simulink model "AB_Final_of_MPC_Bandwidth_Result_UnbalancedNew"  (R2022b)
settings: Solver=FixedStepDiscrete  StartTime=0.0  StopTime=Inf  FixedStep=100e-6  RelTol=1e-3  EnableMultiTasking=on
undefined symbols (not defined in the file): C28x, CPU1, CPU2, CurrentBypassValue, DiscIntNeverNeededParam, Down, GPTRIP1SEL, TZ1, Up
libraries: c2802xlib x20, simulink x17, dspstat3 x13, eeGeneralControl x10, c2837xDlib x5, c280xlib x5, PID_Lib x4, c2000lib x1, spsAlphaBetaZerotoabcLib x1
(part 3 of 10)

== system AB_Final_of_MPC_Bandwidth_Result_UnbalancedNew/Subsystem3 ==
  MPCC_f32GridVoltageA2 : Inport
  MPCC_f32GridVoltageB1 : Inport  Port=2
  MPCC_f32GridVoltageC3 : Inport  Port=3
  function : TriggerPort  TriggerType=function-call  VariantControl=(inherit)
  Add5 : Sum  Inputs=+--
  Cast To Single{,1..4} (5 alike) : DataTypeConversion  OutDataTypeStr=single  SaturateOnIntegerOverflow=off  RndMeth=Floor
  Constant10 : Constant  Value=boolean(0)
  Constant11 : Constant  Value=single(56539)
  Constant12 : Constant  Value=single(100e-6)
  Constant13 : Constant  Value=boolean(0)
  Constant14 : Constant  Value=single(56539)
  Constant15 : Constant  Value=single(100e-6)
  Constant16 : Constant  Value=boolean(0)
  Constant3 : Constant  Value=single(56539)
  Constant4 : Constant  Value=single(100e-6)
  Constant5 : Constant  Value=single(0)
  Constant8 : Constant  Value=36000
  Gain{2,4,8,10} (4 alike) : Gain  Gain=-1
  Gain11 : Gain  Gain=single(1/0.85)
  Gain6 : Gain  Gain=single(1/0.9)
  Gain7 : Gain  Gain=single(1/0.9)
  LPF : Subsystem
  LPF1 : Subsystem
  LPF2 : Subsystem
  PLL_Loop2 : Subsystem
  Rate Limiter Dynamic : simulink/Discontinuities/Rate Limiter Dynamic
  RateLimiter : Subsystem
  RateLimiter1 : Subsystem
  RateLimiter2 : Subsystem
  MPCC_f32AngularFrequency : Outport
  MPCC_f32GridVoltageC : Outport  Port=2
  MPCC_f32ElectricalAngle : Outport  Port=3
  MPCC_f32GridVoltageA : Outport  Port=4
  MPCC_f32GridVoltageB : Outport  Port=5
  wires:
  Cast To Single1/1 -> Gain6/1
  Constant5/1 -> Add5/1
  Cast To Single2/1 -> Gain7/1
  LPF/1(y_k) -> Cast To Single1/1
  LPF2/1(y_k) -> Cast To Single2/1
  Gain7/1 -> Add5/3, PLL_Loop2/2(MPCC_f32GridVoltageB), MPCC_f32GridVoltageB/1
  MPCC_f32GridVoltageA2/1 -> RateLimiter/5(Xo), RateLimiter/4(U), Rate Limiter Dynamic/2
  Constant8/1 -> Gain8/1, Rate Limiter Dynamic/1
  Gain8/1 -> Rate Limiter Dynamic/3
  Constant3/1 -> Gain2/1, RateLimiter/1(Up)
  Gain2/1 -> RateLimiter/3(Lo)
  Constant4/1 -> RateLimiter/2(Ts)
  Constant10/1 -> RateLimiter/6(Rs)
  RateLimiter/1(Y) -> LPF/1(u_k)
  Constant11/1 -> Gain4/1, RateLimiter1/1(Up)
  Constant12/1 -> RateLimiter1/2(Ts)
  Gain4/1 -> RateLimiter1/3(Lo)
  MPCC_f32GridVoltageB1/1 -> RateLimiter1/5(Xo), RateLimiter1/4(U)
  Constant13/1 -> RateLimiter1/6(Rs)
  RateLimiter1/1(Y) -> LPF2/1(u_k)
  RateLimiter2/1(Y) -> LPF1/1(u_k)
  Constant16/1 -> RateLimiter2/6(Rs)
  Gain10/1 -> RateLimiter2/3(Lo)
  Constant15/1 -> RateLimiter2/2(Ts)
  Constant14/1 -> Gain10/1, RateLimiter2/1(Up)
  LPF1/1(y_k) -> Cast To Single4/1
  Cast To Single4/1 -> Gain11/1
  MPCC_f32GridVoltageC3/1 -> RateLimiter2/5(Xo), RateLimiter2/4(U)
  Gain11/1 -> PLL_Loop2/3(MPCC_f32GridVoltageC), MPCC_f32GridVoltageC/1
  PLL_Loop2/1(MPCC_f32AngularFrequency) -> Cast To Single/1
  Gain6/1 -> PLL_Loop2/1(MPCC_f32GridVoltageA), MPCC_f32GridVoltageA/1, Add5/2
  PLL_Loop2/2(MPCC_f32ElectricalAngle) -> Cast To Single3/1
  Cast To Single/1 -> MPCC_f32AngularFrequency/1
  Cast To Single3/1 -> MPCC_f32ElectricalAngle/1

== system AB_Final_of_MPC_Bandwidth_Result_UnbalancedNew/Subsystem4 ==
  function : TriggerPort  TriggerType=function-call  VariantControl=(inherit)
  Constant : Constant  Value=boolean(0)
  Digital Output : c2837xDlib/Digital Output  GPIO_Number=GPIO8~GPIO15  GPIO_Bit0=off  GPIO_BIT0_Toggle=off  GPIO_Bit1=off  GPIO_BIT1_Toggle=off  GPIO_Bit2=off  GPIO_BIT2_Toggle=off  GPIO_Bit3=off  GPIO_BIT3_Toggle=off  GPIO_Bit4=off  GPIO_BIT4_Toggle=off  GPIO_Bit5=off  GPIO_BIT5_Toggle=off  GPIO_Bit6=on  GPIO_BIT6_Toggle=off  GPIO_Bit7=off  GPIO_BIT7_Toggle=off
  wires:
  Constant/1 -> Digital Output/1

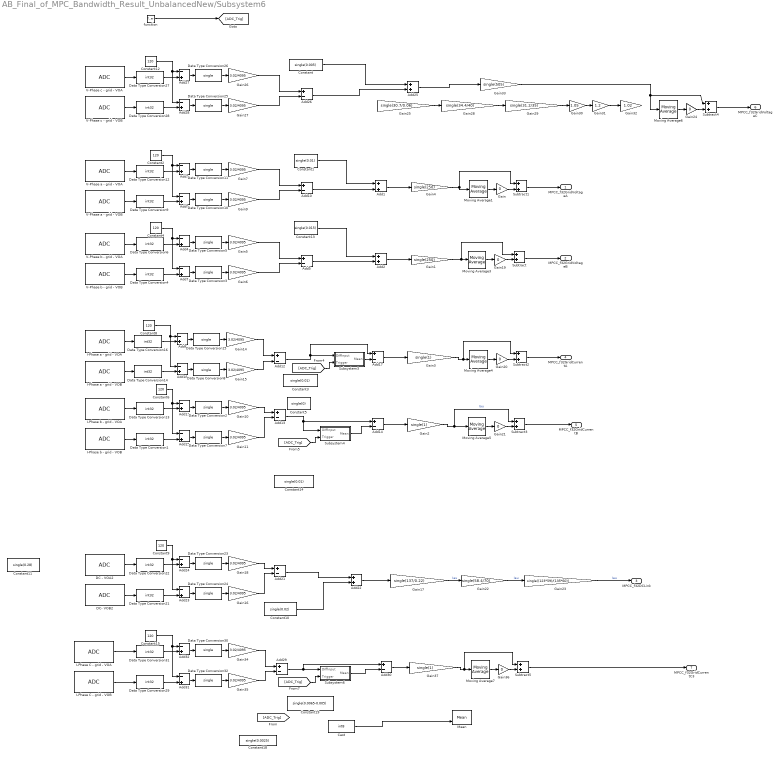
== system AB_Final_of_MPC_Bandwidth_Result_UnbalancedNew/Subsystem6 ==
  function : TriggerPort  TriggerType=function-call  VariantControl=(inherit)  ShowOutputPort=on  OutputDataType=int8
  Add{1..2,22,25} (4 alike) : Sum  AccumDataTypeStr=single  OutDataTypeStr=single
  Add{5,10,12..14,17,21,26,29..30} (10 alike) : Sum  Inputs=+-  AccumDataTypeStr=single  OutDataTypeStr=single
  Add{3..4,6..7,9,11,15,18,23..24,27..28,31..32} (14 alike) : Sum  Inputs=-+  AccumDataTypeStr=single  OutDataTypeStr=single
  Cast : DataTypeConversion  OutDataTypeStr=int8  SaturateOnIntegerOverflow=off  RndMeth=Floor
  Constant : Constant  Value=single(0.005)
  Constant1 : Constant  Value=single(0.01)
  Constant10 : Constant  Value=single(0.02)
  Constant11 : Constant  Value=single(0.28)
  Constant{2,4,6,8..9,12,15} (7 alike) : Constant  Value=120  OutDataTypeStr=single
  Constant13 : Constant  Value=single(0.015)
  Constant14 : Constant  Value=single(0.01)
  Constant18 : Constant  Value=single(0.0025)
  Constant19 : Constant  Value=single(0.0065-0.005)
  Constant3 : Constant  Value=single(0.01)
  Constant5 : Constant  Value=single(0)
  DC - VOA2 : c2802xlib/ADC  blkParamProc=C2000_Type4  ADCModule=C  samplingMode=Single sample mode  ADCResolution=12-bit (Single-ended input)  useSOC1=SOC0  useSOC2=SOC0_SOC1  SOCAcquisitionWindow=22  SOCTriggerSource=ePWM1_ADCSOCA  SOCInterruptTrigger=No ADCINT  Ts=-1  dType=uint16  postInterrupt=off  interruptSel=ADCINT1  ADCINTContinuous=on  endma=off  chdma=1  conv1=ADCINA0  conv2=ADCINA0 and ADCINB0  conv1_Type4=ADCIN5  conv2_Type4=ADCIN0 and ADCIN1
  DC- VOB2 : c2802xlib/ADC  blkParamProc=C2000_Type4  ADCModule=B  samplingMode=Single sample mode  ADCResolution=12-bit (Single-ended input)  useSOC1=SOC3  useSOC2=SOC0_SOC1  SOCAcquisitionWindow=22  SOCTriggerSource=ePWM1_ADCSOCA  SOCInterruptTrigger=No ADCINT  Ts=-1  dType=uint16  postInterrupt=off  interruptSel=ADCINT2  ADCINTContinuous=on  endma=off  chdma=1  conv1=ADCINA0  conv2=ADCINA0 and ADCINB0  conv1_Type4=ADCIN5  conv2_Type4=ADCIN2 and ADCIN3
  Data Type Conversion{1,4,6,9,12..14,16,21..22,27..29,31} (14 alike) : DataTypeConversion  OutDataTypeStr=int32  ConvertRealWorld=Stored Integer (SI)  SaturateOnIntegerOverflow=off  RndMeth=Floor
  Data Type Conversion{2..3,5,7..8,10..11,15,23..26,30,32} (14 alike) : DataTypeConversion  OutDataTypeStr=single  SaturateOnIntegerOverflow=off  RndMeth=Floor
  Gain{,19..21,24,36} (6 alike) : Gain  Gain=0
  Gain1 : Gain  Gain=single(250)
  Gain{5..7,9..11,14..16,18,26..27,34..35} (14 alike) : Gain  Gain=3.02/4095  ParamDataTypeStr=single  OutDataTypeStr=single
  Gain17 : Gain  Gain=single(137/0.22)
  Gain2 : Gain  Gain=single(1)
  Gain22 : Gain  Gain=single(58.4/70)
  Gain23 : Gain  Gain=single((123*59)/(135*60))
  Gain25 : Gain  Gain=single(30.7/0.06)
  Gain28 : Gain  Gain=single(34.4/40)
  Gain29 : Gain  Gain=single(31.2/35)
  Gain3 : Gain  Gain=single(1)
  Gain30 : Gain  Gain=1.05
  Gain31 : Gain  Gain=1.2
  Gain32 : Gain  Gain=1.02
  Gain33 : Gain  Gain=single(505)
  Gain37 : Gain  Gain=single(1)
  Gain4 : Gain  Gain=single(250)
  I-Phase C - grid - VOA : c2802xlib/ADC  blkParamProc=C2000_Type4  ADCModule=A  samplingMode=Single sample mode  ADCResolution=12-bit (Single-ended input)  useSOC1=SOC15  useSOC2=SOC0_SOC1  SOCAcquisitionWindow=22  SOCTriggerSource=ePWM1_ADCSOCA  SOCInterruptTrigger=No ADCINT  Ts=-1  dType=uint16  postInterrupt=off  interruptSel=ADCINT1  ADCINTContinuous=on  endma=off  chdma=1  conv1=ADCINA0  conv2=ADCINA0 and ADCINB0  conv1_Type4=ADCIN15  conv2_Type4=ADCIN0 and ADCIN1
  I-Phase C - grid - VOB : c2802xlib/ADC  blkParamProc=C2000_Type4  ADCModule=A  samplingMode=Single sample mode  ADCResolution=12-bit (Single-ended input)  useSOC1=SOC10  useSOC2=SOC0_SOC1  SOCAcquisitionWindow=22  SOCTriggerSource=ePWM1_ADCSOCA  SOCInterruptTrigger=No ADCINT  Ts=-1  dType=uint16  postInterrupt=off  interruptSel=ADCINT2  ADCINTContinuous=on  endma=off  chdma=1  conv1=ADCINA0  conv2=ADCINA0 and ADCINB0  conv1_Type4=ADCIN14  conv2_Type4=ADCIN2 and ADCIN3
  I-Phase a - grid - VOA : c2802xlib/ADC  blkParamProc=C2000_Type4  ADCModule=A  samplingMode=Single sample mode  ADCResolution=12-bit (Single-ended input)  useSOC1=SOC0  useSOC2=SOC0_SOC1  SOCAcquisitionWindow=22  SOCTriggerSource=ePWM1_ADCSOCA  SOCInterruptTrigger=No ADCINT  Ts=-1  dType=uint16  postInterrupt=on  interruptSel=ADCINT1  ADCINTContinuous=on  endma=off  chdma=1  conv1=ADCINA0  conv2=ADCINA0 and ADCINB0  conv1_Type4=ADCIN4  conv2_Type4=ADCIN0 and ADCIN1
  I-Phase a - grid - VOB : c2802xlib/ADC  blkParamProc=C2000_Type4  ADCModule=B  samplingMode=Single sample mode  ADCResolution=12-bit (Single-ended input)  useSOC1=SOC1  useSOC2=SOC0_SOC1  SOCAcquisitionWindow=22  SOCTriggerSource=ePWM1_ADCSOCA  SOCInterruptTrigger=No ADCINT  Ts=-1  dType=uint16  postInterrupt=off  interruptSel=ADCINT2  ADCINTContinuous=on  endma=off  chdma=1  conv1=ADCINA0  conv2=ADCINA0 and ADCINB0  conv1_Type4=ADCIN4  conv2_Type4=ADCIN2 and ADCIN3
  I-Phase b - grid - VOA : c2802xlib/ADC  blkParamProc=C2000_Type4  ADCModule=C  samplingMode=Single sample mode  ADCResolution=12-bit (Single-ended input)  useSOC1=SOC12  useSOC2=SOC0_SOC1  SOCAcquisitionWindow=22  SOCTriggerSource=ePWM1_ADCSOCA  SOCInterruptTrigger=No ADCINT  Ts=-1  dType=uint16  postInterrupt=off  interruptSel=ADCINT1  ADCINTContinuous=on  endma=off  chdma=1  conv1=ADCINA0  conv2=ADCINA0 and ADCINB0  conv1_Type4=ADCIN4  conv2_Type4=ADCIN0 and ADCIN1
  I-Phase b - grid - VOB : c2802xlib/ADC  blkParamProc=C2000_Type4  ADCModule=A  samplingMode=Single sample mode  ADCResolution=12-bit (Single-ended input)  useSOC1=SOC3  useSOC2=SOC0_SOC1  SOCAcquisitionWindow=22  SOCTriggerSource=ePWM1_ADCSOCA  SOCInterruptTrigger=No ADCINT  Ts=-1  dType=uint16  postInterrupt=off  interruptSel=ADCINT2  ADCINTContinuous=on  endma=off  chdma=1  conv1=ADCINA0  conv2=ADCINA0 and ADCINB0  conv1_Type4=ADCIN5  conv2_Type4=ADCIN2 and ADCIN3
  Mean : dspstat3/Mean  run=on  InputProcessing=Columns as channels (frame based)  reset_popup=Rising edge  directionMode=Each column  dimension=1  roiEnable=off  roiType=Rectangles  roiPortion=Entire ROI  roiOutput=Individual statistics for each ROI  roiFlag=off  roundingMode=Floor  overflowMode=off  outputDataTypeStr=Inherit: Same as accumulator  outputMin=[]  outputMax=[]  outputLastDataTypeStr=Inherit: Same as accumulator
  Moving Average{1,3..7} (6 alike) : dspstat3/Moving Average  Method=Exponential weighting  ForgettingFactorPort=off  SpecifyWindowLength=on  WindowLength=4  OverlapLength=3  AllowArbitraryInputLength=off  ForgettingFactor=0.99  SimulateUsing=Code generation
  Subsystem3 : Subsystem
  Subsystem4 : Subsystem
  Subsystem6 : Subsystem
  Subtract{,1..5} (6 alike) : Sum
  V-Phase a - grid - VOA : c2802xlib/ADC  blkParamProc=C2000_Type4  ADCModule=C  samplingMode=Single sample mode  ADCResolution=12-bit (Single-ended input)  useSOC1=SOC4  useSOC2=SOC0_SOC1  SOCAcquisitionWindow=22  SOCTriggerSource=ePWM1_ADCSOCA  SOCInterruptTrigger=No ADCINT  Ts=-1  dType=uint16  postInterrupt=off  interruptSel=ADCINT1  ADCINTContinuous=on  endma=off  chdma=1  conv1=ADCINA0  conv2=ADCINA0 and ADCINB0  conv1_Type4=ADCIN3  conv2_Type4=ADCIN0 and ADCIN1
  V-Phase a - grid - VOB : c2802xlib/ADC  blkParamProc=C2000_Type4  ADCModule=B  samplingMode=Single sample mode  ADCResolution=12-bit (Single-ended input)  useSOC1=SOC5  useSOC2=SOC0_SOC1  SOCAcquisitionWindow=22  SOCTriggerSource=ePWM1_ADCSOCA  SOCInterruptTrigger=No ADCINT  Ts=-1  dType=uint16  postInterrupt=off  interruptSel=ADCINT2  ADCINTContinuous=on  endma=off  chdma=1  conv1=ADCINA0  conv2=ADCINA0 and ADCINB0  conv1_Type4=ADCIN3  conv2_Type4=ADCIN2 and ADCIN3
  V-Phase b - grid - VOA : c2802xlib/ADC  blkParamProc=C2000_Type4  ADCModule=A  samplingMode=Single sample mode  ADCResolution=12-bit (Single-ended input)  useSOC1=SOC6  useSOC2=SOC0_SOC1  SOCAcquisitionWindow=22  SOCTriggerSource=ePWM1_ADCSOCA  SOCInterruptTrigger=No ADCINT  Ts=-1  dType=uint16  postInterrupt=off  interruptSel=ADCINT1  ADCINTContinuous=on  endma=off  chdma=1  conv1=ADCINA0  conv2=ADCINA0 and ADCINB0  conv1_Type4=ADCIN3  conv2_Type4=ADCIN0 and ADCIN1
  V-Phase b - grid - VOB : c2802xlib/ADC  blkParamProc=C2000_Type4  ADCModule=C  samplingMode=Single sample mode  ADCResolution=12-bit (Single-ended input)  useSOC1=SOC7  useSOC2=SOC0_SOC1  SOCAcquisitionWindow=22  SOCTriggerSource=ePWM1_ADCSOCA  SOCInterruptTrigger=No ADCINT  Ts=-1  dType=uint16  postInterrupt=off  interruptSel=ADCINT2  ADCINTContinuous=on  endma=off  chdma=1  conv1=ADCINA0  conv2=ADCINA0 and ADCINB0  conv1_Type4=ADCIN2  conv2_Type4=ADCIN2 and ADCIN3
  V-Phase c - grid - VOA : c2802xlib/ADC  blkParamProc=C2000_Type4  ADCModule=B  samplingMode=Single sample mode  ADCResolution=12-bit (Single-ended input)  useSOC1=SOC0  useSOC2=SOC0_SOC1  SOCAcquisitionWindow=22  SOCTriggerSource=ePWM1_ADCSOCA  SOCInterruptTrigger=No ADCINT  Ts=-1  dType=uint16  postInterrupt=off  interruptSel=ADCINT1  ADCINTContinuous=on  endma=off  chdma=1  conv1=ADCINA0  conv2=ADCINA0 and ADCINB0  conv1_Type4=ADCIN2  conv2_Type4=ADCIN0 and ADCIN1
  V-Phase c - grid - VOB : c2802xlib/ADC  blkParamProc=C2000_Type4  ADCModule=A  samplingMode=Single sample mode  ADCResolution=12-bit (Single-ended input)  useSOC1=SOC1  useSOC2=SOC0_SOC1  SOCAcquisitionWindow=22  SOCTriggerSource=ePWM1_ADCSOCA  SOCInterruptTrigger=No ADCINT  Ts=-1  dType=uint16  postInterrupt=off  interruptSel=ADCINT2  ADCINTContinuous=on  endma=off  chdma=1  conv1=ADCINA0  conv2=ADCINA0 and ADCINB0  conv1_Type4=ADCIN2  conv2_Type4=ADCIN2 and ADCIN3
  MPCC_f32GridVoltageA : Outport
  MPCC_f32GridVoltageB : Outport  Port=2
  MPCC_f32DCLink : Outport  Port=3
  MPCC_f32GridCurrentA : Outport  Port=4
  MPCC_f32GridCurrentB : Outport  Port=5
  MPCC_f32GridVoltageC : Outport  Port=6
  MPCC_f32GridCurrentC3 : Outport  Port=7
  wires:
  Gain5/1 -> Add5/1
  Data Type Conversion5/1 -> Gain5/1
  Gain1/1 -> Subtract/1, Moving Average3/1
  Add9/1 -> Data Type Conversion10/1
  V-Phase a - grid - VOB/1 -> Data Type Conversion9/1
  Data Type Conversion9/1 -> Add9/2
  Gain7/1 -> Add10/1
  Data Type Conversion10/1 -> Gain9/1
  Data Type Conversion12/1 -> Add3/2
  Add7/1 -> Data Type Conversion3/1
  Data Type Conversion4/1 -> Add7/2
  Data Type Conversion6/1 -> Add4/2
  Gain9/1 -> Add10/2
  V-Phase b - grid - VOB/1 -> Data Type Conversion4/1
  V-Phase b - grid - VOA/1 -> Data Type Conversion6/1
  Add4/1 -> Data Type Conversion5/1
  Add3/1 -> Data Type Conversion11/1
  Data Type Conversion3/1 -> Gain6/1
  Gain6/1 -> Add5/2
  Constant4/1 -> Add7/1, Add4/1
  V-Phase a - grid - VOA/1 -> Data Type Conversion12/1
  Constant2/1 -> Add9/1, Add3/1
  Data Type Conversion11/1 -> Gain7/1
  Add1/1 -> Gain4/1
  Add2/1 -> Gain1/1
  I-Phase b - grid - VOA/1 -> Data Type Conversion13/1
  Data Type Conversion15/1 -> Gain14/1
  Data Type Conversion8/1 -> Gain15/1
  Data Type Conversion14/1 -> Add18/2
  Gain15/1 -> Add12/2
  Data Type Conversion13/1 -> Add11/2
  Data Type Conversion16/1 -> Add6/2
  Gain14/1 -> Add12/1
  Add6/1 -> Data Type Conversion15/1
  Gain10/1 -> Add13/1
  Add18/1 -> Data Type Conversion8/1
  I-Phase a - grid - VOA/1 -> Data Type Conversion16/1
  Gain2/1 -> Subtract3/1, Moving Average5/1  "Iau"
  Data Type Conversion2/1 -> Gain10/1
  Constant6/1 -> Add15/1, Add11/1
  I-Phase b - grid - VOB/1 -> Data Type Conversion1/1
  Data Type Conversion1/1 -> Add15/2
  Gain11/1 -> Add13/2
  Add17/1 -> Gain3/1
  Add11/1 -> Data Type Conversion2/1
  Constant8/1 -> Add18/1, Add6/1
  I-Phase a - grid - VOB/1 -> Data Type Conversion14/1
  Data Type Conversion7/1 -> Gain11/1
  Add15/1 -> Data Type Conversion7/1
  Subtract/1 -> MPCC_f32GridVoltageB/1
  Moving Average3/1 -> Gain19/1
  Moving Average1/1 -> Gain/1
  Gain4/1 -> Subtract1/1, Moving Average1/1
  Subtract1/1 -> MPCC_f32GridVoltageA/1
  Moving Average4/1 -> Gain20/1
  Gain3/1 -> Subtract2/1, Moving Average4/1
  Moving Average5/1 -> Gain21/1
  Data Type Conversion22/1 -> Add24/2
  DC- VOB2/1 -> Data Type Conversion21/1
  Data Type Conversion21/1 -> Add23/2
  Data Type Conversion23/1 -> Gain18/1
  DC - VOA2/1 -> Data Type Conversion22/1
  Add24/1 -> Data Type Conversion23/1
  Constant9/1 -> Add23/1, Add24/1
  Gain16/1 -> Add21/2
  Add23/1 -> Data Type Conversion24/1
  Data Type Conversion24/1 -> Gain16/1
  Gain18/1 -> Add21/1
  Gain/1 -> Subtract1/2
  Gain19/1 -> Subtract/2
  Gain20/1 -> Subtract2/2
  Gain21/1 -> Subtract3/2
  Gain17/1 -> Gain22/1  "Iau"
  Subtract2/1 -> MPCC_f32GridCurrentA/1
  Subtract3/1 -> MPCC_f32GridCurrentB/1
  Gain22/1 -> Gain23/1  "Iau"
  V-Phase c - grid - VOB/1 -> Data Type Conversion28/1
  Gain26/1 -> Add26/1
  Data Type Conversion25/1 -> Gain27/1
  V-Phase c - grid - VOA/1 -> Data Type Conversion27/1
  Subtract4/1 -> MPCC_f32GridVoltageC/1
  Data Type Conversion26/1 -> Gain26/1
  Data Type Conversion27/1 -> Add27/2
  Moving Average6/1 -> Gain24/1
  Data Type Conversion28/1 -> Add28/2
  Gain27/1 -> Add26/2
  Add28/1 -> Data Type Conversion25/1
  Constant12/1 -> Add28/1, Add27/1
  Add27/1 -> Data Type Conversion26/1
  Gain25/1 -> Gain28/1
  Gain24/1 -> Subtract4/2
  Gain28/1 -> Gain29/1
  Gain29/1 -> Gain30/1
  Gain30/1 -> Gain31/1
  Gain31/1 -> Gain32/1
  Gain33/1 -> Subtract4/1, Moving Average6/1
  Add31/1 -> Data Type Conversion32/1
  Data Type Conversion32/1 -> Gain35/1
  Data Type Conversion31/1 -> Add32/2
  Gain34/1 -> Add29/1
  Constant15/1 -> Add31/1, Add32/1
  Gain35/1 -> Add29/2
  Subtract5/1 -> MPCC_f32GridCurrentC3/1
  Gain36/1 -> Subtract5/2
  Data Type Conversion30/1 -> Gain34/1
  Data Type Conversion29/1 -> Add31/2
  I-Phase C - grid - VOB/1 -> Data Type Conversion29/1
  I-Phase C - grid - VOA/1 -> Data Type Conversion31/1
  Gain37/1 -> Subtract5/1, Moving Average7/1
  Add32/1 -> Data Type Conversion30/1
  Add30/1 -> Gain37/1
  Moving Average7/1 -> Gain36/1
  Add22/1 -> Gain17/1
  Add14/1 -> Gain2/1
  function/1 -> [ADC_Trig]
  Cast/1 -> Mean/2
  Add25/1 -> Gain33/1
  [ADC_Trig] -> Subsystem3/2(Trigger)
  Add12/1 -> Add17/1, Subsystem3/1(DiffInput)
  Subsystem3/1(Mean) -> Add17/2
  [ADC_Trig] -> Subsystem4/2(Trigger)
  Add13/1 -> Add14/1, Subsystem4/1(DiffInput)
  Subsystem4/1(Mean) -> Add14/2
  [ADC_Trig] -> Subsystem6/2(Trigger)
  Add29/1 -> Add30/1, Subsystem6/1(DiffInput)
  Subsystem6/1(Mean) -> Add30/2
  Constant/1 -> Add25/1
  Add26/1 -> Add25/2
  Constant1/1 -> Add1/1
  Add10/1 -> Add1/2
  Constant13/1 -> Add2/1
  Add5/1 -> Add2/2
  Gain23/1 -> MPCC_f32DCLink/1  "Iau"
  Add21/1 -> Add22/1
  Constant10/1 -> Add22/2

== system AB_Final_of_MPC_Bandwidth_Result_UnbalancedNew/Voltage_Loop ==
  PI_f32DCLinkVoltageRef : Inport
  PI_f32DCLinkVoltage : Inport  Port=2
  PI_f32DCLink : Inport  Port=3
  VoltageLoop_FC : TriggerPort  TriggerType=function-call  VariantControl=(inherit)  SampleTime=-1
      settings: AttributesFormatString=|
      | %<StatesWhenEnabling>
      | %<SampleTime>
  Add : Sum  Inputs=+-
  Cast To Single : DataTypeConversion  OutDataTypeStr=single  SaturateOnIntegerOverflow=off  RndMeth=Floor
  Cast To Single1 : DataTypeConversion  OutDataTypeStr=single  SaturateOnIntegerOverflow=off  RndMeth=Floor
  Cast To Single3 : DataTypeConversion  OutDataTypeStr=single  SaturateOnIntegerOverflow=off  RndMeth=Floor
  Constant : Constant  Commented=on  Value=single(0.2)
  Constant1 : Constant  Commented=on  Value=single(10)
  Constant10 : Constant  Value=single(2.2)
  Constant11 : Constant  Value=single(0.03111)
  Constant12 : Constant  Value=single(0.8685252)
  Constant13 : Constant  Value=single(0.01955)
  Constant2 : Constant  Value=single(7/7)
  Constant3 : Constant  Value=boolean(1)
  Constant4 : Constant  Value=boolean(0)
  Constant5 : Constant  Value=boolean(1)
  Constant6 : Constant  Value=single(0.2)
  Constant7 : Constant  Value=single(0)
  Constant8 : Constant  Commented=on  Value=CurrentBypassValue
  Constant9 : Constant  Value=single(10)
  Gain : Gain  Gain=-1
  Gain1 : Gain  Gain=single(7)
  Gain2 : Gain  Gain=1/300
  Gain3 : Gain  Gain=1/300
  Mux2 : Mux  Inputs=3
  PI : PID_Lib/PI  SystemSampleTime=-1  VariantActivationTime=update diagram  Latency=0  AutoFrameSizeCalculation=off
  Scope : Scope
  Step : Step  Time=30  Before=-0.5  After=-1.5
  Subsystem5 : Subsystem  Commented=through
  Switch : Switch  Criteria=u2 ~= 0  SaturateOnIntegerOverflow=off  InputSameDT=off
  Terminator{,1..4} (5 alike) : Terminator
  PI_f32DGridCurrentReference : Outport
  MPCC_f32DCLinkFiltered : Outport  Port=2
  MPCC_f32DCLinkref : Outport  Port=3
  wires:
  Constant2/1 -> Gain/1, PI/4
  Gain/1 -> PI/5
  Constant3/1 -> PI/6
  Constant4/1 -> PI/7
  PI/2 -> Terminator/1
  PI/3 -> Terminator1/1
  PI/4 -> Terminator2/1
  PI/5 -> Terminator3/1
  Constant5/1 -> Switch/2
  PI/1 -> Switch/1, Scope/1
  Switch/1 -> Cast To Single/1
  Cast To Single1/1 -> Gain2/1
  Cast To Single/1 -> Gain1/1
  Cast To Single3/1 -> Gain3/1, MPCC_f32DCLinkref/1
  PI_f32DCLinkVoltage/1 -> Subsystem5/1(MPCC_f32DCLink)
  Subsystem5/1(MPCC_f32DCLinkFiltered) -> MPCC_f32DCLinkFiltered/1, Cast To Single1/1
  Constant7/1 -> PI/8
  Step/1 -> Switch/3
  Add/1 -> Mux2/1, PI/1
  Gain1/1 -> Mux2/2, PI_f32DGridCurrentReference/1
  Gain3/1 -> Add/1
  Gain2/1 -> Add/2
  PI_f32DCLink/1 -> Mux2/3
  PI_f32DCLinkVoltageRef/1 -> Cast To Single3/1
  Mux2/1 -> Terminator4/1
  Constant6/1 -> PI/2
  Constant9/1 -> PI/3

== system AB_Final_of_MPC_Bandwidth_Result_UnbalancedNew/Subsystem1/ABCtoAlphaBeta ==
  In1 : Inport
  In2 : Inport  Port=2
  In3 : Inport  Port=3
  Add : Sum  Inputs=+-
  Add1 : Sum  Inputs=+--
  Gain : Gain  Gain=0.5
  Gain1 : Gain  Gain=sqrt(3)/2
  Gain2 : Gain  Gain=2/3
  Gain3 : Gain  Gain=2/3
  Gain4 : Gain  Gain=0.5
  alpha : Outport
  Vαβ : Outport  Port=2
  wires:
  In1/1 -> Add1/1
  Gain4/1 -> Add1/3
  Gain/1 -> Add1/2
  In2/1 -> Add/1, Gain/1
  In3/1 -> Add/2, Gain4/1
  Add/1 -> Gain1/1
  Add1/1 -> Gain2/1
  Gain2/1 -> alpha/1
  Gain1/1 -> Gain3/1
  Gain3/1 -> Vαβ/1

== system AB_Final_of_MPC_Bandwidth_Result_UnbalancedNew/Subsystem1/ABCtoD ==
  MPCC_f32DGridCurrent : Inport
  MPCC_f32QGridCurrent : Inport  Port=2
  MPCC_f32ElectricalAngle : Inport  Port=3
  Add : Sum  Inputs=+-
  Cast To Single : DataTypeConversion  OutDataTypeStr=single  SaturateOnIntegerOverflow=off  RndMeth=Floor
  Gain1 : Gain  Gain=2
  LPF : Subsystem
  LPF1 : Subsystem
  Low-Pass Filter (Discrete or Continuous)3 : eeGeneralControl/Low-Pass Filter (Discrete or Continuous)  Commented=on  K=1  T=1/(2*pi*100)  B=inf  A=-inf  init_option=Inherited from block input  x0=0  Ts=-1
  Product : Product
  Product1 : Product
  Sin1 : Trigonometry
  Sin3 : Trigonometry  Operator=cos
  MPCC_f32HarmonicDGridCurrent : Outport
  wires:
  Sin1/1 -> Product1/2
  MPCC_f32ElectricalAngle/1 -> Gain1/1
  Product1/1 -> Add/2
  Product/1 -> Add/1
  [MPCC_f32ElectricalAngle] -> Sin1/1
  MPCC_f32QGridCurrent/1 -> Product1/1
  [MPCC_f32ElectricalAngle] -> Sin3/1
  MPCC_f32DGridCurrent/1 -> Product/1
  Sin3/1 -> Product/2
  Gain1/1 -> [MPCC_f32ElectricalAngle]
  Add/1 -> Cast To Single/1
  Cast To Single/1 -> MPCC_f32HarmonicDGridCurrent/1

== system AB_Final_of_MPC_Bandwidth_Result_UnbalancedNew/Subsystem1/ABCtoD1Pos ==
  MPCC_f32DGridCurrent : Inport
  MPCC_f32QGridCurrent : Inport  Port=2
  MPCC_f32ElectricalAngle : Inport  Port=3
  Add : Sum
  Cast To Single : DataTypeConversion  OutDataTypeStr=single  SaturateOnIntegerOverflow=off  RndMeth=Floor
  Gain : Gain
  Gain1 : Gain  Gain=-2
  LPF : Subsystem
  LPF1 : Subsystem
  LPF2 : Subsystem
  Low-Pass Filter (Discrete or Continuous)3 : eeGeneralControl/Low-Pass Filter (Discrete or Continuous)  Commented=on  K=1  T=1/(2*pi*100)  B=inf  A=-inf  init_option=Inherited from block input  x0=0  Ts=-1
  Product : Product
  Product1 : Product
  Sin1 : Trigonometry
  Sin3 : Trigonometry  Operator=cos
  MPCC_f32HarmonicDGridCurrent : Outport
  wires:
  Sin1/1 -> Product1/2
  MPCC_f32ElectricalAngle/1 -> Gain1/1
  Product1/1 -> Add/2
  Product/1 -> Add/1
  [MPCC_f32ElectricalAngle] -> Sin1/1
  MPCC_f32QGridCurrent/1 -> Product1/1
  [MPCC_f32ElectricalAngle] -> Sin3/1
  MPCC_f32DGridCurrent/1 -> Product/1
  Sin3/1 -> Product/2
  Gain1/1 -> [MPCC_f32ElectricalAngle]
  Add/1 -> LPF2/1(u_k)
  LPF2/1(y_k) -> Gain/1
  Cast To Single/1 -> MPCC_f32HarmonicDGridCurrent/1
  Gain/1 -> Cast To Single/1

== system AB_Final_of_MPC_Bandwidth_Result_UnbalancedNew/Subsystem1/ABCtoD1Pos1 ==
  MPCC_f32DGridCurrent : Inport
  MPCC_f32QGridCurrent : Inport  Port=2
  MPCC_f32ElectricalAngle : Inport  Port=3
  Add : Sum
  Cast To Single : DataTypeConversion  OutDataTypeStr=single  SaturateOnIntegerOverflow=off  RndMeth=Floor
  Gain1 : Gain  Gain=-2
  LPF : Subsystem
  LPF1 : Subsystem
  LPF2 : Subsystem
  Low-Pass Filter (Discrete or Continuous)3 : eeGeneralControl/Low-Pass Filter (Discrete or Continuous)  Commented=on  K=1  T=1/(2*pi*100)  B=inf  A=-inf  init_option=Inherited from block input  x0=0  Ts=-1
  Product : Product
  Product1 : Product
  Sin1 : Trigonometry
  Sin3 : Trigonometry  Operator=cos
  MPCC_f32HarmonicDGridCurrent : Outport
  wires:
  Sin1/1 -> Product1/2
  MPCC_f32ElectricalAngle/1 -> Gain1/1
  Product1/1 -> Add/2
  Product/1 -> Add/1
  [MPCC_f32ElectricalAngle] -> Sin1/1
  MPCC_f32QGridCurrent/1 -> Product1/1
  [MPCC_f32ElectricalAngle] -> Sin3/1
  MPCC_f32DGridCurrent/1 -> Product/1
  Sin3/1 -> Product/2
  Gain1/1 -> [MPCC_f32ElectricalAngle]
  Add/1 -> LPF2/1(u_k)
  LPF2/1(y_k) -> Cast To Single/1
  Cast To Single/1 -> MPCC_f32HarmonicDGridCurrent/1

== system AB_Final_of_MPC_Bandwidth_Result_UnbalancedNew/Subsystem1/ABCtoD1Pos2 ==
  MPCC_f32DGridCurrent : Inport
  MPCC_f32QGridCurrent : Inport  Port=2
  MPCC_f32ElectricalAngle : Inport  Port=3
  Add : Sum
  Cast To Single : DataTypeConversion  OutDataTypeStr=single  SaturateOnIntegerOverflow=off  RndMeth=Floor
  Gain : Gain
  Gain1 : Gain  Gain=-1
  LPF : Subsystem
  LPF1 : Subsystem
  LPF2 : Subsystem
  Low-Pass Filter (Discrete or Continuous)3 : eeGeneralControl/Low-Pass Filter (Discrete or Continuous)  Commented=on  K=1  T=1/(2*pi*100)  B=inf  A=-inf  init_option=Inherited from block input  x0=0  Ts=-1
  Product : Product
  Product1 : Product
  Sin1 : Trigonometry
  Sin3 : Trigonometry  Operator=cos
  MPCC_f32HarmonicDGridCurrent : Outport
  wires:
  Sin1/1 -> Product1/2
  MPCC_f32ElectricalAngle/1 -> Gain1/1
  Product1/1 -> Add/2
  Product/1 -> Add/1
  [MPCC_f32ElectricalAngle] -> Sin1/1
  MPCC_f32QGridCurrent/1 -> Product1/1
  [MPCC_f32ElectricalAngle] -> Sin3/1
  MPCC_f32DGridCurrent/1 -> Product/1
  Sin3/1 -> Product/2
  Gain1/1 -> [MPCC_f32ElectricalAngle]
  Add/1 -> LPF2/1(u_k)
  LPF2/1(y_k) -> Gain/1
  Cast To Single/1 -> MPCC_f32HarmonicDGridCurrent/1
  Gain/1 -> Cast To Single/1

== system AB_Final_of_MPC_Bandwidth_Result_UnbalancedNew/Subsystem1/ABCtoD2 ==
  MPCC_f32DGridCurrent : Inport
  MPCC_f32QGridCurrent : Inport  Port=2
  MPCC_f32ElectricalAngle : Inport  Port=3
  Add : Sum  Inputs=+-
  Cast To Single : DataTypeConversion  OutDataTypeStr=single  SaturateOnIntegerOverflow=off  RndMeth=Floor
  Gain1 : Gain  Gain=-2
  LPF : Subsystem
  LPF1 : Subsystem
  Low-Pass Filter (Discrete or Continuous)3 : eeGeneralControl/Low-Pass Filter (Discrete or Continuous)  Commented=on  K=1  T=1/(2*pi*100)  B=inf  A=-inf  init_option=Inherited from block input  x0=0  Ts=-1
  Product : Product
  Product1 : Product
  Sin1 : Trigonometry
  Sin3 : Trigonometry  Operator=cos
  MPCC_f32HarmonicDGridCurrent : Outport
  wires:
  Sin1/1 -> Product1/2
  MPCC_f32ElectricalAngle/1 -> Gain1/1
  Product1/1 -> Add/2
  Product/1 -> Add/1
  [MPCC_f32ElectricalAngle] -> Sin1/1
  MPCC_f32QGridCurrent/1 -> Product1/1
  [MPCC_f32ElectricalAngle] -> Sin3/1
  MPCC_f32DGridCurrent/1 -> Product/1
  Sin3/1 -> Product/2
  Gain1/1 -> [MPCC_f32ElectricalAngle]
  Add/1 -> Cast To Single/1
  Cast To Single/1 -> MPCC_f32HarmonicDGridCurrent/1

== system AB_Final_of_MPC_Bandwidth_Result_UnbalancedNew/Subsystem1/ABCtoD2Neg ==
  MPCC_f32DGridCurrent : Inport
  MPCC_f32QGridCurrent : Inport  Port=2
  MPCC_f32ElectricalAngle : Inport  Port=3
  Add : Sum  Inputs=-+
  Cast To Single : DataTypeConversion  OutDataTypeStr=single  SaturateOnIntegerOverflow=off  RndMeth=Floor
  Gain : Gain
  Gain1 : Gain  Gain=2
  LPF : Subsystem
  LPF1 : Subsystem
  LPF2 : Subsystem
  Low-Pass Filter (Discrete or Continuous)3 : eeGeneralControl/Low-Pass Filter (Discrete or Continuous)  Commented=on  K=1  T=1/(2*pi*100)  B=inf  A=-inf  init_option=Inherited from block input  x0=0  Ts=-1
  Product : Product
  Product1 : Product
  Sin1 : Trigonometry  Operator=cos
  Sin3 : Trigonometry
  MPCC_f32HarmonicDGridCurrent : Outport
  wires:
  Sin1/1 -> Product1/2
  MPCC_f32ElectricalAngle/1 -> Gain1/1
  Product1/1 -> Add/2
  Product/1 -> Add/1
  [MPCC_f32ElectricalAngle] -> Sin1/1
  MPCC_f32QGridCurrent/1 -> Product1/1
  [MPCC_f32ElectricalAngle] -> Sin3/1
  MPCC_f32DGridCurrent/1 -> Product/1
  Sin3/1 -> Product/2
  Gain1/1 -> [MPCC_f32ElectricalAngle]
  Add/1 -> LPF2/1(u_k)
  LPF2/1(y_k) -> Gain/1
  Cast To Single/1 -> MPCC_f32HarmonicDGridCurrent/1
  Gain/1 -> Cast To Single/1

== system AB_Final_of_MPC_Bandwidth_Result_UnbalancedNew/Subsystem1/ABCtoD2Neg1 ==
  MPCC_f32DGridCurrent : Inport
  MPCC_f32QGridCurrent : Inport  Port=2
  MPCC_f32ElectricalAngle : Inport  Port=3
  Add : Sum  Inputs=-+
  Cast To Single : DataTypeConversion  OutDataTypeStr=single  SaturateOnIntegerOverflow=off  RndMeth=Floor
  Gain1 : Gain  Gain=-2
  LPF : Subsystem
  LPF1 : Subsystem
  LPF2 : Subsystem
  Low-Pass Filter (Discrete or Continuous)3 : eeGeneralControl/Low-Pass Filter (Discrete or Continuous)  Commented=on  K=1  T=1/(2*pi*100)  B=inf  A=-inf  init_option=Inherited from block input  x0=0  Ts=-1
  Product : Product
  Product1 : Product
  Sin1 : Trigonometry  Operator=cos
  Sin3 : Trigonometry
  MPCC_f32HarmonicDGridCurrent : Outport
  wires:
  Sin1/1 -> Product1/2
  MPCC_f32ElectricalAngle/1 -> Gain1/1
  Product1/1 -> Add/2
  Product/1 -> Add/1
  [MPCC_f32ElectricalAngle] -> Sin1/1
  MPCC_f32QGridCurrent/1 -> Product1/1
  [MPCC_f32ElectricalAngle] -> Sin3/1
  MPCC_f32DGridCurrent/1 -> Product/1
  Sin3/1 -> Product/2
  Gain1/1 -> [MPCC_f32ElectricalAngle]
  Add/1 -> LPF2/1(u_k)
  LPF2/1(y_k) -> Cast To Single/1
  Cast To Single/1 -> MPCC_f32HarmonicDGridCurrent/1

== system AB_Final_of_MPC_Bandwidth_Result_UnbalancedNew/Subsystem1/ABCtoD3 ==
  MPCC_f32DGridCurrent : Inport
  MPCC_f32QGridCurrent : Inport  Port=2
  MPCC_f32ElectricalAngle : Inport  Port=3
  Add : Sum  Inputs=+-
  Cast To Single : DataTypeConversion  OutDataTypeStr=single  SaturateOnIntegerOverflow=off  RndMeth=Floor
  Gain1 : Gain  Gain=-2
  LPF : Subsystem
  LPF1 : Subsystem
  Low-Pass Filter (Discrete or Continuous)3 : eeGeneralControl/Low-Pass Filter (Discrete or Continuous)  Commented=on  K=1  T=1/(2*pi*100)  B=inf  A=-inf  init_option=Inherited from block input  x0=0  Ts=-1
  Product : Product
  Product1 : Product
  Sin1 : Trigonometry
  Sin3 : Trigonometry  Operator=cos
  MPCC_f32HarmonicDGridCurrent : Outport
  wires:
  Sin1/1 -> Product1/2
  MPCC_f32ElectricalAngle/1 -> Gain1/1
  Product1/1 -> Add/2
  Product/1 -> Add/1
  [MPCC_f32ElectricalAngle] -> Sin1/1
  MPCC_f32QGridCurrent/1 -> Product1/1
  [MPCC_f32ElectricalAngle] -> Sin3/1
  MPCC_f32DGridCurrent/1 -> Product/1
  Sin3/1 -> Product/2
  Gain1/1 -> [MPCC_f32ElectricalAngle]
  Add/1 -> Cast To Single/1
  Cast To Single/1 -> MPCC_f32HarmonicDGridCurrent/1

== system AB_Final_of_MPC_Bandwidth_Result_UnbalancedNew/Subsystem1/ABCtoDQO ==
  PI_f32GridCurrentA : Inport
  PI_f32GridCurrentB : Inport  Port=2
  PI_f32GridCurrentC : Inport  Port=3
  PI_f32GridVoltageA : Inport  Port=4
  PI_f32GridVoltageB : Inport  Port=5
  PI_f32GridVoltageC : Inport  Port=6
  PI_f32ElectricalAngle : Inport  Port=7
  Cast To Single : DataTypeConversion  OutDataTypeStr=single  SaturateOnIntegerOverflow=off  RndMeth=Floor
  Cast To Single1 : DataTypeConversion  OutDataTypeStr=single  SaturateOnIntegerOverflow=off  RndMeth=Floor
  Ground : Ground
  abc_dq : Subsystem
  abc_dq1 : Subsystem
  PI_f32DGridCurrent : Outport
  PI_f32QGridCurrent : Outport  Port=2
  PI_f32OGridCurrent : Outport  Port=3
  PI_f32DGridVoltage : Outport  Port=4
  PI_f32QGridVoltage : Outport  Port=5
  PI_f32OGridVoltage : Outport  Port=6
  wires:
  abc_dq/1(Id) -> Cast To Single/1
  abc_dq/2(Iq) -> Cast To Single1/1
  PI_f32ElectricalAngle/1 -> [PI_f32ElectricalAngle]
  Ground/1 -> PI_f32OGridCurrent/1, PI_f32OGridVoltage/1
  abc_dq1/2(Iq) -> PI_f32QGridVoltage/1
  [PI_f32ElectricalAngle] -> ?
  abc_dq1/1(Id) -> PI_f32DGridVoltage/1
  PI_f32GridCurrentC/1 -> abc_dq/3(c)
  PI_f32GridCurrentB/1 -> abc_dq/2(b)
  PI_f32GridCurrentA/1 -> abc_dq/1(a)
  PI_f32GridVoltageA/1 -> abc_dq1/1(a)
  PI_f32GridVoltageB/1 -> abc_dq1/2(b)
  PI_f32GridVoltageC/1 -> abc_dq1/3(c)
  Cast To Single/1 -> PI_f32DGridCurrent/1
  Cast To Single1/1 -> PI_f32QGridCurrent/1

== system AB_Final_of_MPC_Bandwidth_Result_UnbalancedNew/Subsystem1/ABCtoQ ==
  MPCC_f32DGridCurrent : Inport
  MPCC_f32QGridCurrent : Inport  Port=2
  MPCC_f32ElectricalAngle : Inport  Port=3
  Add : Sum
  Cast To Single : DataTypeConversion  OutDataTypeStr=single  SaturateOnIntegerOverflow=off  RndMeth=Floor
  Gain1 : Gain  Gain=-2
  LPF : Subsystem  Commented=on
  LPF1 : Subsystem
  LPF2 : Subsystem  Commented=on
  LPF3 : Subsystem
  Low-Pass Filter (Discrete or Continuous)3 : eeGeneralControl/Low-Pass Filter (Discrete or Continuous)  Commented=on  K=1  T=1/(2*pi*100)  B=inf  A=-inf  init_option=Inherited from block input  x0=0  Ts=-1
  Product : Product
  Product1 : Product
  Sin1 : Trigonometry  Operator=cos
  Sin3 : Trigonometry
  MPCC_f32HarmonicQGridCurrent : Outport
  wires:
  Sin1/1 -> Product1/2
  MPCC_f32ElectricalAngle/1 -> Gain1/1
  Product1/1 -> Add/2
  Product/1 -> Add/1
  [MPCC_f32ElectricalAngle] -> Sin1/1
  MPCC_f32QGridCurrent/1 -> Product1/1
  [MPCC_f32ElectricalAngle] -> Sin3/1
  MPCC_f32DGridCurrent/1 -> Product/1
  Sin3/1 -> Product/2
  Gain1/1 -> [MPCC_f32ElectricalAngle]
  Add/1 -> Cast To Single/1
  Cast To Single/1 -> MPCC_f32HarmonicQGridCurrent/1

== system AB_Final_of_MPC_Bandwidth_Result_UnbalancedNew/Subsystem1/ABCtoQPos1 ==
  MPCC_f32DGridCurrent : Inport
  MPCC_f32QGridCurrent : Inport  Port=2
  MPCC_f32ElectricalAngle : Inport  Port=3
  Add : Sum  Inputs=-+
  Cast To Single : DataTypeConversion  OutDataTypeStr=single  SaturateOnIntegerOverflow=off  RndMeth=Floor
  Gain1 : Gain  Gain=-2
  LPF : Subsystem
  LPF1 : Subsystem
  LPF2 : Subsystem
  Low-Pass Filter (Discrete or Continuous)3 : eeGeneralControl/Low-Pass Filter (Discrete or Continuous)  Commented=on  K=1  T=1/(2*pi*100)  B=inf  A=-inf  init_option=Inherited from block input  x0=0  Ts=-1
  Product : Product
  Product1 : Product
  Sin1 : Trigonometry  Operator=cos
  Sin3 : Trigonometry
  MPCC_f32HarmonicQGridCurrent : Outport
  wires:
  Sin1/1 -> Product1/2
  MPCC_f32ElectricalAngle/1 -> Gain1/1
  Product1/1 -> Add/2
  Product/1 -> Add/1
  [MPCC_f32ElectricalAngle] -> Sin1/1
  MPCC_f32QGridCurrent/1 -> Product1/1
  [MPCC_f32ElectricalAngle] -> Sin3/1
  MPCC_f32DGridCurrent/1 -> Product/1
  Sin3/1 -> Product/2
  Gain1/1 -> [MPCC_f32ElectricalAngle]
  Add/1 -> LPF2/1(u_k)
  LPF2/1(y_k) -> Cast To Single/1
  Cast To Single/1 -> MPCC_f32HarmonicQGridCurrent/1

== system AB_Final_of_MPC_Bandwidth_Result_UnbalancedNew/Subsystem1/AlphaBetaDutiesCalculation ==
  MPCC_f32DVoltageReference : Inport
  MPCC_f32QVoltageReference : Inport  Port=2
  MPCC_f32ElectricalAngle_K_1 : Inport  Port=3
  MPCC_f32DCLinkVoltage : Inport  Port=4
  AlphaBetaVoltageReferenceCalculation : Subsystem
  DutiesCalculation : Subsystem
  MPCC_f32AlphaVoltageReference : Outport
  MPCC_f32BetaVoltageReference : Outport  Port=2
  MPCC_f32Duty_Sector1 : Outport  Port=3
  MPCC_f32Duty_Sector2 : Outport  Port=4
  MPCC_f32Duty_Sector3 : Outport  Port=5
  MPCC_f32Duty_Sector4 : Outport  Port=6
  MPCC_f32Duty_Sector5 : Outport  Port=7
  MPCC_f32Duty_Sector6 : Outport  Port=8
  wires:
  MPCC_f32ElectricalAngle_K_1/1 -> AlphaBetaVoltageReferenceCalculation/3(MPCC_f32ElectricalAngle_K_1)
  AlphaBetaVoltageReferenceCalculation/1(MPCC_f32AlphaVoltageReference) -> MPCC_f32AlphaVoltageReference/1
  AlphaBetaVoltageReferenceCalculation/2(MPCC_f32BetaVoltageReference) -> MPCC_f32BetaVoltageReference/1
  DutiesCalculation/1(MPCC_f32Duty_Sector1) -> MPCC_f32Duty_Sector1/1
  DutiesCalculation/2(MPCC_f32Duty_Sector2) -> MPCC_f32Duty_Sector2/1
  DutiesCalculation/3(MPCC_f32Duty_Sector3) -> MPCC_f32Duty_Sector3/1
  DutiesCalculation/4(MPCC_f32Duty_Sector4) -> MPCC_f32Duty_Sector4/1
  DutiesCalculation/6(MPCC_f32Duty_Sector6) -> MPCC_f32Duty_Sector6/1
  DutiesCalculation/5(MPCC_f32Duty_Sector5) -> MPCC_f32Duty_Sector5/1
  MPCC_f32DCLinkVoltage/1 -> DutiesCalculation/3(MPCC_f32DCLinkVoltage)
  [MPCC_f32AlphaVoltageReference] -> DutiesCalculation/1(MPCC_f32AlphaVoltageReference)
  [MPCC_f32BetaVoltageReference] -> DutiesCalculation/2(MPCC_f32BetaVoltageReference)
  MPCC_f32DVoltageReference/1 -> [MPCC_f32AlphaVoltageReference]
  MPCC_f32QVoltageReference/1 -> [MPCC_f32BetaVoltageReference]

== system AB_Final_of_MPC_Bandwidth_Result_UnbalancedNew/Subsystem1/AlphaBetaVoltageReferenceCalculation ==
  MPCC_f32DVoltageReference : Inport
  MPCC_f32QVoltageReference : Inport  Port=2
  MPCC_f32ElectricalAngle_K_1 : Inport  Port=3
  Add : Sum  Inputs=+-
  Add1 : Sum
  Product{,1..3} (4 alike) : Product
  Sin : Trigonometry  Operator=cos
  Sin1 : Trigonometry
  Sin2 : Trigonometry
  Sin3 : Trigonometry  Operator=cos
  MPCC_f32AlphaVoltageReference : Outport
  MPCC_f32BetaVoltageReference : Outport  Port=2
  wires:
  Sin2/1 -> Product2/1
  [MPCC_f32QVoltageReference] -> Product3/2
  Sin1/1 -> Product1/1
  Sin3/1 -> Product3/1
  Product/1 -> Add/1
  [MPCC_f32DVoltageReference] -> Product2/2
  [MPCC_f32ElectricalAngle_K_1] -> Sin2/1
  [MPCC_f32QVoltageReference] -> Product1/2
  Add1/1 -> MPCC_f32BetaVoltageReference/1
  Product2/1 -> Add1/1
  Product3/1 -> Add1/2
  [MPCC_f32ElectricalAngle_K_1] -> Sin3/1
  MPCC_f32DVoltageReference/1 -> [MPCC_f32DVoltageReference]
  Add/1 -> MPCC_f32AlphaVoltageReference/1
  [MPCC_f32ElectricalAngle_K_1] -> Sin/1
  [MPCC_f32DVoltageReference] -> Product/2
  MPCC_f32QVoltageReference/1 -> [MPCC_f32QVoltageReference]
  Product1/1 -> Add/2
  Sin/1 -> Product/1
  [MPCC_f32ElectricalAngle_K_1] -> Sin1/1
  MPCC_f32ElectricalAngle_K_1/1 -> [MPCC_f32ElectricalAngle_K_1]

== system AB_Final_of_MPC_Bandwidth_Result_UnbalancedNew/Subsystem1/AlphaBetaVoltageReferenceCalculation1 ==
  MPCC_f32DVoltageReference : Inport
  MPCC_f32QVoltageReference : Inport  Port=2
  MPCC_f32ElectricalAngle_K_1 : Inport  Port=3
  Add : Sum  Inputs=+-
  Add1 : Sum
  Product{,1..3} (4 alike) : Product
  Sin : Trigonometry  Operator=cos
  Sin1 : Trigonometry
  Sin2 : Trigonometry
  Sin3 : Trigonometry  Operator=cos
  MPCC_f32AlphaVoltageReference : Outport
  MPCC_f32BetaVoltageReference : Outport  Port=2
  wires:
  Sin2/1 -> Product2/1
  [MPCC_f32QVoltageReference] -> Product3/2
  Sin1/1 -> Product1/1
  Sin3/1 -> Product3/1
  Product/1 -> Add/1
  [MPCC_f32DVoltageReference] -> Product2/2
  [MPCC_f32ElectricalAngle_K_1] -> Sin2/1
  [MPCC_f32QVoltageReference] -> Product1/2
  Add1/1 -> MPCC_f32BetaVoltageReference/1
  Product2/1 -> Add1/1
  Product3/1 -> Add1/2
  [MPCC_f32ElectricalAngle_K_1] -> Sin3/1
  MPCC_f32DVoltageReference/1 -> [MPCC_f32DVoltageReference]
  Add/1 -> MPCC_f32AlphaVoltageReference/1
  [MPCC_f32ElectricalAngle_K_1] -> Sin/1
  [MPCC_f32DVoltageReference] -> Product/2
  MPCC_f32QVoltageReference/1 -> [MPCC_f32QVoltageReference]
  Product1/1 -> Add/2
  Sin/1 -> Product/1
  [MPCC_f32ElectricalAngle_K_1] -> Sin1/1
  MPCC_f32ElectricalAngle_K_1/1 -> [MPCC_f32ElectricalAngle_K_1]

== system AB_Final_of_MPC_Bandwidth_Result_UnbalancedNew/Subsystem1/Angle_Identification  ==
  A : Inport
  B : Inport  Port=2
  C : Inport  Port=3
  Fcn : Fcn  Expr=(u(1)-0.5*u(2)-0.5*u(3))
  Fcn2 : Fcn  Expr=((sqrt(3)/2)*(u(2)))-((sqrt(3)/2)*(u(3)))
  Gain : Gain  Gain=2/3
  Gain1 : Gain  Gain=2/3
  Mux : Mux  Inputs=3
  V_alpha : Outport
  V_beta : Outport  Port=2
  wires:
  C/1 -> Mux/3
  A/1 -> Mux/1
  B/1 -> Mux/2
  Mux/1 -> Fcn2/1, Fcn/1
  Fcn/1 -> Gain1/1
  Fcn2/1 -> Gain/1
  Gain1/1 -> V_alpha/1
  Gain/1 -> V_beta/1

== system AB_Final_of_MPC_Bandwidth_Result_UnbalancedNew/Subsystem1/CodeGeneration1 ==
  Input : Inport
  Add : Sum  Inputs=+-  OutDataTypeStr=Inherit: Same as first input
  Demux2 : Demux  Outputs=2
  Index Vector : MultiPortSwitch  Inputs=1  SaturateOnIntegerOverflow=off  InputSameDT=off
  SCI Transmit : c280xlib/SCI Transmit  sciModule=A  dataHead=''  dataTail=''  blockingMode=on  outputStatus=off
  While Iterator : WhileIterator  MaxIters=-1  WhileBlockType=do-while  ShowIterationPort=on  OutputDataType=int16
  wires:
  While Iterator/1 -> Add/2, Index Vector/1
  Demux2/1 -> Index Vector/2
  Index Vector/1 -> SCI Transmit/1
  Add/1 -> While Iterator/1
  Demux2/2 -> Add/1
  Input/1 -> Demux2/1

== system AB_Final_of_MPC_Bandwidth_Result_UnbalancedNew/Subsystem1/Data1 ==
  Data : Inport
  Data_width : Inport  Port=2
  Action Port : ActionPort  ActionPortLabel=else
  Mux : Mux  Inputs=2
  Start : Constant  Value=hex2dec('0000')  OutDataTypeStr=uint16
  Data_out : Outport  VectorParamsAs1DForOutWhenUnconnected=off
  Iteration : Outport  Port=2  VectorParamsAs1DForOutWhenUnconnected=off
  wires:
  Start/1 -> Mux/2
  Mux/1 -> Data_out/1
  Data/1 -> Mux/1
  Data_width/1 -> Iteration/1

== system AB_Final_of_MPC_Bandwidth_Result_UnbalancedNew/Subsystem1/Data_Conditioning1 ==
  In1 : Inport
  Data Type Conversion3 : DataTypeConversion  OutDataTypeStr=uint16  ConvertRealWorld=Stored Integer (SI)  SaturateOnIntegerOverflow=off  RndMeth=Floor
  Out1 : Outport  VectorParamsAs1DForOutWhenUnconnected=off
  wires:
  Data Type Conversion3/1 -> Out1/1
  In1/1 -> Data Type Conversion3/1

== system AB_Final_of_MPC_Bandwidth_Result_UnbalancedNew/Subsystem1/Decoupling_Loop ==
  PI_f32DGridCurrent : Inport
  PI_f32QGridCurrent : Inport  Port=2
  PI_f32DGridVoltage : Inport  Port=3
  PI_f32QGridVoltage : Inport  Port=4
  PI_f32AngularFrequency : Inport  Port=5
  PI_f32DCLinkVoltage : Inport  Port=6
  PI_f32LGrid : Inport  Port=7
  PI_f32DVoltage : Inport  Port=8
  PI_f32QVoltage : Inport  Port=9
  PI_f32ElectricalAngle : Inport  Port=10
  ABCtoDQOVoltage : Subsystem  Commented=on
  Cast To Single : DataTypeConversion  OutDataTypeStr=single  SaturateOnIntegerOverflow=off  RndMeth=Floor
  Cast To Single1 : DataTypeConversion  OutDataTypeStr=single  SaturateOnIntegerOverflow=off  RndMeth=Floor
  Cast To Single2 : DataTypeConversion  OutDataTypeStr=single  SaturateOnIntegerOverflow=off  RndMeth=Floor
  Constant : Constant  Value=single(0)
  Decoupling_Loop : Subsystem
  Saturation : Saturate  UpperLimit=single(2/sqrt(3))  LowerLimit=single(-2/sqrt(3))
  Saturation1 : Saturate  UpperLimit=single(2/sqrt(3))  LowerLimit=single(-2/sqrt(3))
  Terminator : Terminator
  dq_abc : Subsystem
  PI_f32MAVoltageRef : Outport
  PI_f32MBVoltageRef : Outport  Port=2
  PI_f32MCVoltageRef : Outport  Port=3
  wires:
  PI_f32DGridCurrent/1 -> Decoupling_Loop/1(PI_f32DGridCurrent)
  PI_f32QGridCurrent/1 -> Decoupling_Loop/2(PI_f32QGridCurrent)
  PI_f32DGridVoltage/1 -> Decoupling_Loop/3(PI_f32DGridVoltage)
  PI_f32QGridVoltage/1 -> Decoupling_Loop/4(PI_f32QGridVoltage)
  PI_f32AngularFrequency/1 -> Decoupling_Loop/5(PI_f32AngularFrequency)
  PI_f32LGrid/1 -> Decoupling_Loop/7(PI_f32LGrid)
  PI_f32DVoltage/1 -> Decoupling_Loop/8(PI_f32DVoltage)
  PI_f32QVoltage/1 -> Decoupling_Loop/9(PI_f32QVoltage)
  PI_f32ElectricalAngle/1 -> [PI_f32ElectricalAngle]
  Decoupling_Loop/1(PI_f32MDVoltageRef) -> Saturation/1
  Decoupling_Loop/2(PI_f32MQVoltageRef) -> Saturation1/1
  PI_f32DCLinkVoltage/1 -> Decoupling_Loop/6(PI_f32DCLinkVoltage)
  [PI_f32ElectricalAngle] -> dq_abc/1(theta)
  Constant/1 -> Terminator/1
  [PI_f32MDVoltageRef] -> dq_abc/2(vd)
  [PI_f32MQVoltageRef] -> dq_abc/3(vq)
  dq_abc/2(Ib) -> Cast To Single1/1
  dq_abc/3(Ic) -> Cast To Single2/1
  dq_abc/1(Ia) -> Cast To Single/1
  Saturation/1 -> [PI_f32MDVoltageRef]
  Saturation1/1 -> [PI_f32MQVoltageRef]
  Cast To Single/1 -> PI_f32MAVoltageRef/1
  Cast To Single1/1 -> PI_f32MBVoltageRef/1
  Cast To Single2/1 -> PI_f32MCVoltageRef/1

== system AB_Final_of_MPC_Bandwidth_Result_UnbalancedNew/Subsystem1/End1 ==
  Data : Inport
  Data_width : Inport  Port=2
  Action Port : ActionPort  ActionPortLabel=elseif(u1 == 599)
  Bias : Bias  Bias=1  SaturateOnIntegerOverflow=off
  Mux : Mux  Inputs=2
  Start : Constant  Value=hex2dec('4545')  OutDataTypeStr=uint16
  Data_out : Outport  VectorParamsAs1DForOutWhenUnconnected=off
  Iteration : Outport  Port=2  VectorParamsAs1DForOutWhenUnconnected=off
  wires:
  Mux/1 -> Data_out/1
  Data_width/1 -> Bias/1
  Start/1 -> Mux/2
  Bias/1 -> Iteration/1
  Data/1 -> Mux/1

== system AB_Final_of_MPC_Bandwidth_Result_UnbalancedNew/Subsystem1/GridCurrentFirstPrediction ==
  MPCC_f32Predictionterm_A : Inport
  MPCC_f32Predictionterm_B : Inport  Port=2
  MPCC_f32Predictionterm_C : Inport  Port=3
  MPCC_f32DGridCurrent : Inport  Port=4
  MPCC_f32QGridCurrent : Inport  Port=5
  MPCC_f32DGridVoltage : Inport  Port=6
  MPCC_f32QGridVoltage : Inport  Port=7
  MPCC_f32DConvVoltage : Inport  Port=8
  MPCC_f32QConvVoltage : Inport  Port=9
  PredictedIdGridCurrentCalculation : Subsystem
  PredictedIqGridCurrentCalculation : Subsystem
  MPCC_f32DGridCurrent_K_1 : Outport
  MPCC_f32QGridCurrent_K_1 : Outport  Port=2
  wires:
  MPCC_f32DGridVoltage/1 -> [MPCC_f32DGridVoltage]
  MPCC_f32Predictionterm_A/1 -> [MPCC_f32Predictionterm_A]
  MPCC_f32QGridVoltage/1 -> [MPCC_f32QGridVoltage]
  MPCC_f32Predictionterm_C/1 -> [MPCC_f32Predictionterm_C]
  MPCC_f32Predictionterm_B/1 -> [MPCC_f32Predictionterm_B]
  MPCC_f32DGridCurrent/1 -> [MPCC_f32DGridCurrent]
  MPCC_f32QGridCurrent/1 -> [MPCC_f32QGridCurrent]
  PredictedIdGridCurrentCalculation/1(MPCC_f32DGridCurrent_K_1) -> MPCC_f32DGridCurrent_K_1/1
  PredictedIqGridCurrentCalculation/1(MPCC_f32QVoltageReference) -> MPCC_f32QGridCurrent_K_1/1
  [MPCC_f32Predictionterm_A] -> PredictedIdGridCurrentCalculation/1(MPCC_f32Predictionterm_A)
  [MPCC_f32Predictionterm_B] -> PredictedIdGridCurrentCalculation/2(MPCC_f32Predictionterm_B)
  [MPCC_f32Predictionterm_C] -> PredictedIdGridCurrentCalculation/3(MPCC_f32Predictionterm_C)
  [MPCC_f32DGridCurrent] -> PredictedIdGridCurrentCalculation/4(MPCC_f32DGridCurrent)
  [MPCC_f32QGridCurrent] -> PredictedIdGridCurrentCalculation/5(MPCC_f32QGridCurrent)
  [MPCC_f32DGridVoltage] -> PredictedIdGridCurrentCalculation/6(MPCC_f32DGridVoltage)
  [MPCC_f32DConvVoltage] -> PredictedIdGridCurrentCalculation/7(MPCC_f32DConvVoltage)
  MPCC_f32DConvVoltage/1 -> [MPCC_f32DConvVoltage]
  MPCC_f32QConvVoltage/1 -> [MPCC_f32QConvVoltage]
  [MPCC_f32Predictionterm_A] -> PredictedIqGridCurrentCalculation/1(MPCC_f32Predictionterm_A)
  [MPCC_f32Predictionterm_C] -> PredictedIqGridCurrentCalculation/3(MPCC_f32Predictionterm_C)
  [MPCC_f32QGridCurrent] -> PredictedIqGridCurrentCalculation/5(MPCC_f32QGridCurrent)
  [MPCC_f32QGridVoltage] -> PredictedIqGridCurrentCalculation/6(MPCC_f32QGridVoltage)
  [MPCC_f32QConvVoltage] -> PredictedIqGridCurrentCalculation/7(MPCC_f32QConvVoltage)
  [MPCC_f32Predictionterm_B] -> PredictedIqGridCurrentCalculation/2(MPCC_f32Predictionterm_B)
  [MPCC_f32DGridCurrent] -> PredictedIqGridCurrentCalculation/4(MPCC_f32DGridCurrent)
